simulink model "SimulinkLineTracking"  (R2019b)
settings: Solver=FixedStepAuto  StartTime=0.0  StopTime=14  RelTol=1e-3  EnableMultiTasking=on
libraries: legoev3lib x9, simulink x1
settings Model: ExtModeTrigDuration=1  Creator=nikit  LastModifiedBy=nikit
settings SolverCC: PositivePriorityOrder=on
settings OptimizationCC: EnhancedBackFolding=on  PassReuseOutputArgsAs=Individual arguments  ZeroExternalMemoryAtStartup=off  ZeroInternalMemoryAtStartup=off  MaxStackSize=64  OptimizeBlockOrder=speed  DifferentSizesBufferReuse=on  EfficientTunableParamExpr=on
settings DebuggingCC: ParameterTunabilityLossMsg=error
settings HardwareCC: ProdBitPerPointer=32  ProdBitPerSizeT=32  ProdBitPerPtrDiffT=32  ProdLargestAtomicInteger=Long  ProdWordSize=32  ProdHWDeviceType=ARM Compatible->ARM 9
settings SFSimCC: MATLABDynamicMemAlloc=off
settings RTWCC: SystemTargetFile=ert.tlc  HardwareBoard=LEGO MINDSTORMS EV3  TLCOptions="-aInlineSetEventsForThisBaseRateFcn=TLC_FALSE -aSuppressMultiTaskScheduler=TLC_FALSE  -aRateBasedStepFcn=0"  TemplateMakefile=ert_default_tmf  GenerateReport=on  Toolchain=Sourcery G++ Lite v2009q3  IncludeHyperlinkInReport=on  LaunchReport=on  GenerateTraceInfo=on  GenerateTraceReport=on  GenerateTraceReportSl=on  GenerateTraceReportSf=on  GenerateTraceReportEml=on
settings CodeAppCC: ForceParamTrailComments=on  IgnoreCustomStorageClasses=off  OperatorAnnotations=on  SimulinkDataObjDesc=on  SFDataObjDesc=on  InsertBlockDesc=on
settings ERTTargetCC: SupportContinuousTime=on  SupportVariableSizeSignals=on

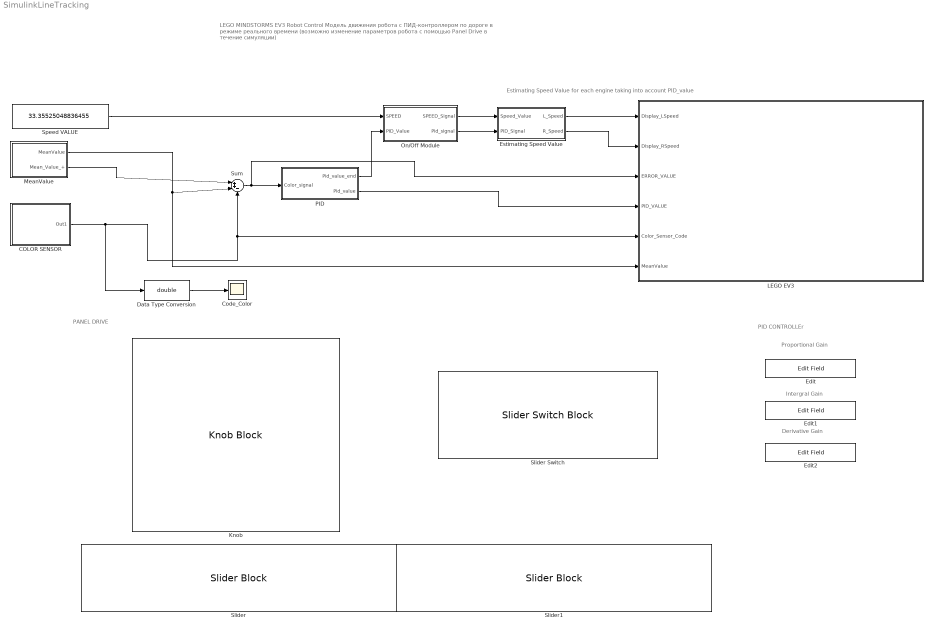
== system SimulinkLineTracking ==
  note: PID CONTROLLEr
  note: Derivative Gain
  note: Estimating Speed Value for each engine taking into account PID_value
  note: PANEL DRIVE
  note: Proportional Gain
  note: Intergral Gain
  note: LEGO MINDSTORMS EV3 Robot Control
      | Модель движения робота с ПИД-контроллером по дороге в режиме реального времени
      | (возможно изменение параметров робота с помощью Panel Drive в течение симуляции)
  COLOR SENSOR : Subsystem
  Code_Color : Scope
  Data Type Conversion : DataTypeConversion  OutDataTypeStr=double
  Edit : EditField  LabelPosition=Hide  ShowInitialText=on  Alignment=Center
  Edit1 : EditField  LabelPosition=Hide  ShowInitialText=on  Alignment=Center
  Edit2 : EditField  LabelPosition=Hide  ShowInitialText=on  Alignment=Center
  Estimating Speed Value : Subsystem
  Knob : KnobBlock
  "LEGO EV3 " : Subsystem
      mask Display: image('C:\Users\nikit\Desktop\ev3-robot-educator-color-sensor-down-39f06f3533b0bf031fff0c5aebbdd482.jpg'); % Use "Edit Image" on toolstrip to change.
  MeanValue : Subsystem
  "On/Off Module " : Subsystem
  PID : Subsystem
  Slider : SliderBlock  ScaleMin=-20  ScaleMax=20
  Slider Switch : SliderSwitchBlock
      settings: Values={{'Off', 'On'}, [0 1]}
  Slider1 : SliderBlock  ScaleMin=-10  ScaleMax=10
  "Speed VALUE\t" : Constant  Value=33.35525048836455  OutDataTypeStr=int8
  Sum : Sum  Inputs=|++-
  wires:
  Sum/1 -> "LEGO EV3 "/3(ERROR_VALUE), PID/1(Color_signal)
  COLOR SENSOR/1(Out1) -> Data Type Conversion/1, Sum/3, "LEGO EV3 "/5(Color_Sensor_Code)
  Data Type Conversion/1 -> Code_Color/1
  Estimating Speed Value/1(L_Speed) -> "LEGO EV3 "/1(Display_LSpeed)
  Estimating Speed Value/2(R_Speed) -> "LEGO EV3 "/2(Display_RSpeed)
  "Speed VALUE\t"/1 -> "On/Off Module "/1(SPEED)
  "On/Off Module "/1(SPEED_Signal) -> Estimating Speed Value/1(Speed_Value)
  "On/Off Module "/2(Pid_signal) -> Estimating Speed Value/2(PID_Signal)
  PID/1(Pid_value_end) -> "On/Off Module "/2(PID_Value)
  PID/2(Pid_value) -> "LEGO EV3 "/4(PID_VALUE)
  MeanValue/1(MeanValue) -> "LEGO EV3 "/6(MeanValue), Sum/2
  MeanValue/2(Mean_Value_+) -> Sum/1

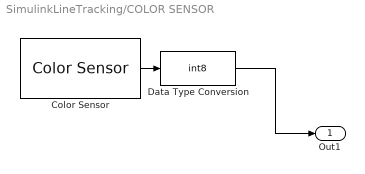
== system SimulinkLineTracking/COLOR SENSOR ==
  Color Sensor : legoev3lib/Color Sensor  portNumber=2  mode=Reflected light intensity  sampleTime=0.01
      settings: SourceProductName=Simulink Support Package for LEGO MINDSTORMS EV3 Hardware  SourceProductBaseCode=LEGOEV3
  Data Type Conversion : DataTypeConversion  OutDataTypeStr=int8
  Out1 : Outport
  wires:
  Color Sensor/1 -> Data Type Conversion/1
  Data Type Conversion/1 -> Out1/1

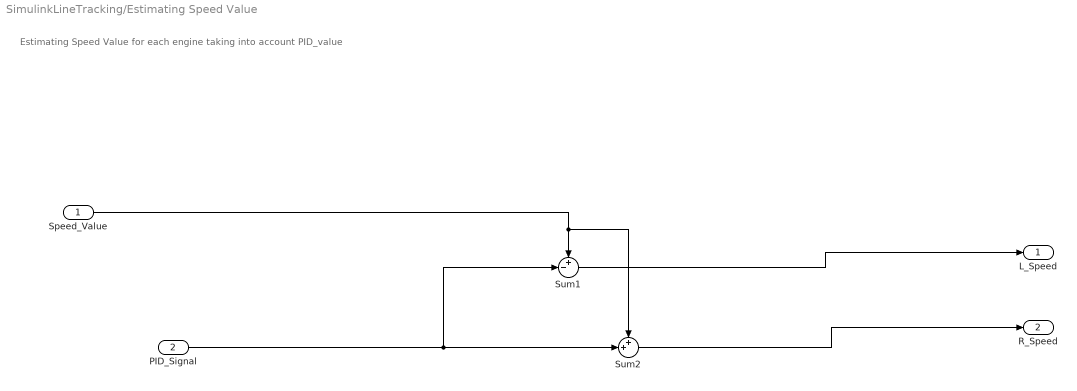
== system SimulinkLineTracking/Estimating Speed Value ==
  note: Estimating Speed Value for each engine taking into account PID_value
  Speed_Value : Inport
  PID_Signal : Inport  Port=2
  Sum1 : Sum  Inputs=+-|
  Sum2 : Sum  Inputs=++|
  L_Speed : Outport
  R_Speed : Outport  Port=2
  wires:
  Speed_Value/1 -> Sum2/1, Sum1/1
  PID_Signal/1 -> Sum2/2, Sum1/2
  Sum2/1 -> R_Speed/1
  Sum1/1 -> L_Speed/1

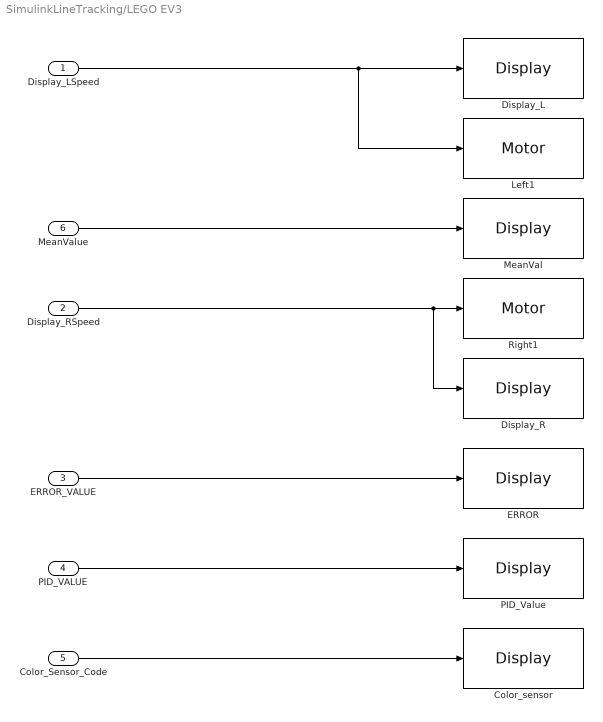
== system SimulinkLineTracking/LEGO EV3  ==
  Display_LSpeed : Inport
  Display_RSpeed : Inport  Port=2
  ERROR_VALUE : Inport  Port=3
  PID_VALUE : Inport  Port=4
  Color_Sensor_Code : Inport  Port=5
  MeanValue : Inport  Port=6
  Color_sensor : legoev3lib/Display  slcdStr=Color  slcdLine=3  slcdFormat=Decimal
      settings: SourceProductName=Simulink Support Package for LEGO MINDSTORMS EV3 Hardware  SourceProductBaseCode=LEGOEV3
  Display_L : legoev3lib/Display  slcdStr=Left  slcdLine=1  slcdFormat=Decimal
      settings: SourceProductName=Simulink Support Package for LEGO MINDSTORMS EV3 Hardware  SourceProductBaseCode=LEGOEV3
  Display_R : legoev3lib/Display  slcdStr=Right  slcdLine=2  slcdFormat=Decimal
      settings: SourceProductName=Simulink Support Package for LEGO MINDSTORMS EV3 Hardware  SourceProductBaseCode=LEGOEV3
  ERROR : legoev3lib/Display  slcdStr=Error  slcdLine=4  slcdFormat=Decimal
      settings: SourceProductName=Simulink Support Package for LEGO MINDSTORMS EV3 Hardware  SourceProductBaseCode=LEGOEV3
  Left1 : legoev3lib/Motor  sportNumber=A  sstopAction=Brake
  MeanVal : legoev3lib/Display  slcdStr=MeanVal  slcdLine=6  slcdFormat=Decimal
      settings: SourceProductName=Simulink Support Package for LEGO MINDSTORMS EV3 Hardware  SourceProductBaseCode=LEGOEV3
  PID_Value : legoev3lib/Display  slcdStr=PID  slcdLine=5  slcdFormat=Decimal
      settings: SourceProductName=Simulink Support Package for LEGO MINDSTORMS EV3 Hardware  SourceProductBaseCode=LEGOEV3
  Right1 : legoev3lib/Motor  sportNumber=D  sstopAction=Brake
  wires:
  ERROR_VALUE/1 -> ERROR/1
  MeanValue/1 -> MeanVal/1
  Display_LSpeed/1 -> Left1/1, Display_L/1
  Color_Sensor_Code/1 -> Color_sensor/1
  Display_RSpeed/1 -> Display_R/1, Right1/1
  PID_VALUE/1 -> PID_Value/1

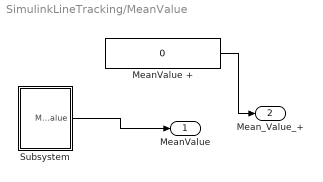
== system SimulinkLineTracking/MeanValue ==
  MeanValue + : Constant  Value=0  OutDataTypeStr=int8
  Subsystem : Subsystem  mask(Find mean value of two colors){Black=3, White=45}
      mask prompts: Black "BlackColorCode"; White "WhiteColorCode"
      mask help: You need to write codes of two colors to find mean value
  MeanValue : Outport
  Mean_Value_+ : Outport  Port=2
  wires:
  Subsystem/1(MeanValue) -> MeanValue/1
  MeanValue +/1 -> Mean_Value_+/1

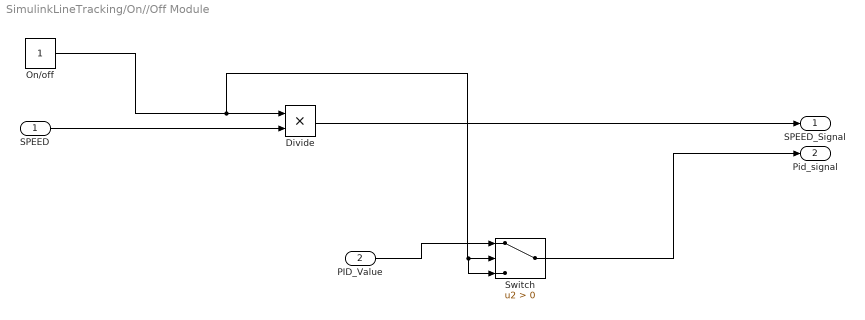
== system SimulinkLineTracking/On//Off Module  ==
  SPEED : Inport
  PID_Value : Inport  Port=2
  Divide : Product  Inputs=**
  On/off : Constant  OutDataTypeStr=int8
  Switch : Switch  Criteria=u2 > Threshold
  SPEED_Signal : Outport
  Pid_signal : Outport  Port=2
  wires:
  On/off/1 -> Switch/3, Switch/2, Divide/1
  Switch/1 -> Pid_signal/1
  SPEED/1 -> Divide/2
  Divide/1 -> SPEED_Signal/1
  PID_Value/1 -> Switch/1

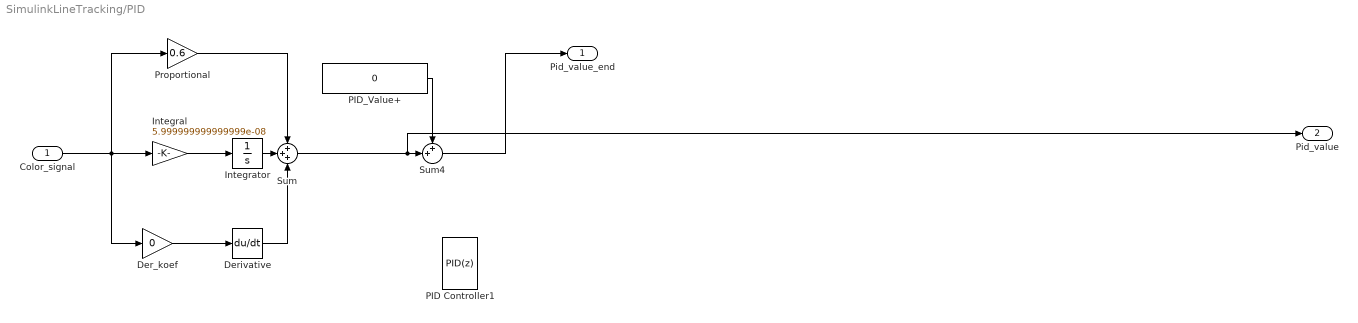
== system SimulinkLineTracking/PID ==
  Color_signal : Inport
  Der_koef : Gain  Gain=0
  Derivative : Derivative
  Integral : Gain  Gain=5.999999999999999e-08
  Integrator : Integrator
  PID Controller1 : simulink/Continuous/PID Controller  Controller=PID  Form=Parallel  TimeDomain=Discrete-time  SampleTime=-1  IntegratorMethod=Forward Euler  FilterMethod=Forward Euler  ControllerParametersSource=internal  P=0.6  I=0.00000006  D=0  UseFilter=on  N=100  TunerSelectOption=Transfer Function Based (PID Tuner App)  InitialConditionSource=internal  InitialConditionForIntegrator=0  InitialConditionForFilter=0  DifferentiatorICPrevScaledInput=0  ExternalReset=none  TrackingMode=off  Kt=1  LimitOutput=off  UpperSaturationLimit=inf  LowerSaturationLimit=-inf  LinearizeAsGain=on  AntiWindupMode=none  Kb=1  POutMin=[]  POutMax=[]  IOutMin=[]  IOutMax=[]  DOutMin=[]  DOutMax=[]  NOutMin=[]  NOutMax=[]  SumOutMin=[]  SumOutMax=[]  SaturationOutMin=[]  SaturationOutMax=[]  PParamMin=[]  PParamMax=[]  IParamMin=[]  IParamMax=[]  DParamMin=[]  DParamMax=[]  NParamMin=[]  NParamMax=[]  KbParamMin=[]  KbParamMax=[]  KtParamMin=[]  KtParamMax=[]  KbOutMin=[]  KbOutMax=[]  KtOutMin=[]  KtOutMax=[]  IntegratorOutMin=[]  IntegratorOutMax=[]  FilterOutMin=[]  FilterOutMax=[]  SumI1OutMin=[]  SumI1OutMax=[]  SumI2OutMin=[]  SumI2OutMax=[]  SumI3OutMin=[]  SumI3OutMax=[]  SumI4OutMin=[]  SumI4OutMax=[]  SumDOutMin=[]  SumDOutMax=[]  DifferentiatorOutMin=[]  DifferentiatorOutMax=[]  FilterDiffOutCoefMin=[]  FilterDiffOutCoefMax=[]  ReciprocalOutMin=[]  ReciprocalOutMax=[]  SumDenOutMin=[]  SumDenOutMax=[]  SumNumOutMin=[]  SumNumOutMax=[]  DivideOutMin=[]  DivideOutMax=[]  IntegratorContinuousStateAttributes=''  IntegratorStateMustResolveToSignalObject=off  IntegratorRTWStateStorageClass=Auto  FilterContinuousStateAttributes=''  FilterStateMustResolveToSignalObject=off  FilterRTWStateStorageClass=Auto  ParallelPVariant=InternalParameters  IdealPVariant=Disabled  IVariant=InternalParameters  DVariant=InternalParameters  IntegratorVariant=Discrete  SatVariant=Disabled  AWVariant=Passthrough  PCopyVariant=Disabled  TRVariant=Disabled  FdbkBlocksVariant=Forward  IdealPFdbkVariant=Disabled  SatFdbkVariant=Disabled  DerivativeFilterVariant=ForwardEulerFilter  NVariant=InternalParameters  NCopyVariant=Disabled  FilterICVariant=InternalICsFilter  IntegratorICVariant=InternalICs  ExternalResetVariant=Disabled  TRSumVariant=Passthrough  SumFdbkVariant=Disabled  SumVariant=Sum_PID
  PID_Value+ : Constant  Value=0  OutDataTypeStr=int8
  Proportional : Gain  Gain=0.6
  Sum : Sum  Inputs=+++
  Sum4 : Sum  Inputs=++|
  Pid_value_end : Outport
  Pid_value : Outport  Port=2
  wires:
  Sum4/1 -> Pid_value_end/1
  PID_Value+/1 -> Sum4/1
  Sum/1 -> Pid_value/1, Sum4/2
  Color_signal/1 -> Integral/1, Der_koef/1, Proportional/1
  Integrator/1 -> Sum/2
  Derivative/1 -> Sum/3
  Der_koef/1 -> Derivative/1
  Proportional/1 -> Sum/1
  Integral/1 -> Integrator/1

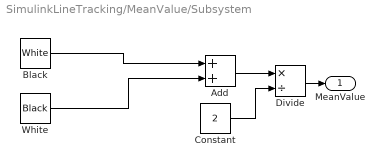
== system SimulinkLineTracking/MeanValue/Subsystem ==
  Add : Sum  OutDataTypeStr=int8
  Black : Constant  Value=White
  Constant : Constant  Value=2
  Divide : Product  Inputs=*/
  White : Constant  Value=Black
  MeanValue : Outport
  wires:
  Add/1 -> Divide/1
  Constant/1 -> Divide/2
  White/1 -> Add/2
  Divide/1 -> MeanValue/1
  Black/1 -> Add/1
